simulink model "Tonneau"  (R2023b)
settings: Solver=VariableStepAuto  StartTime=0.0  StopTime=60  RelTol=1e-3
values from neighbouring files (symbols this model uses):
  p = @(t)  interp1(     [0, t_fin/30, t_fin/10, t_fin/5, 0.7*t_fin, 0.9*t_fin, t_fin],     [0, p_max/40, p_max*3/4,  p_max,     p_max,         0,     0],     t, 'pchip'  )    [ESERCIZIO_3_3.m]    (also in main.m = @(t)      interp1(          [0 t_fin/30 t_fin/10 t_fin/5 0.7; plotTrajectoryAndBody.m = patch('faces', F, 'vertices' ,Vb))
  PosE0 = [X0;Y0;Z0]    [ESERCIZIO_3_3.m]    (also in main.m = [0;0;0])
  Q0 = angle2quat(psi0, theta0, phi0)    [ESERCIZIO_3_3.m]    (also in main.m)
libraries: aerolibconvert2 x2, sharedtransform x2, SignalEditorBlockLib x2, aerolibutil x1
settings Model: Creator=Vincenzo  LastModifiedBy=agode
settings SolverCC: AlgebraicLoopSolver=TrustRegion
settings DebuggingCC: UnconnectedInputMsg=warning  UnconnectedOutputMsg=warning  UnconnectedLineMsg=warning  ArithmeticOperatorsInVariantConditions=warning
settings ModelReferenceCC: EnableRefExpFcnMdlSchedulingChecks=on
settings SFSimCC: SimUseLocalCustomCode=off  CustomCodeUndefinedFunction=UseInterfaceOnly
settings RTWCC: RTWUseLocalCustomCode=off

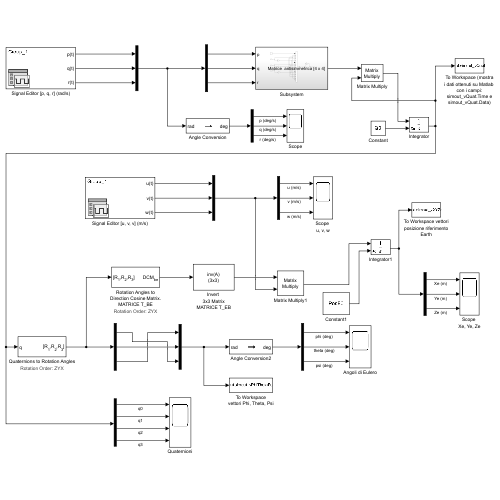
[thumbnail: Simulink's stored preview of the top-level diagram]
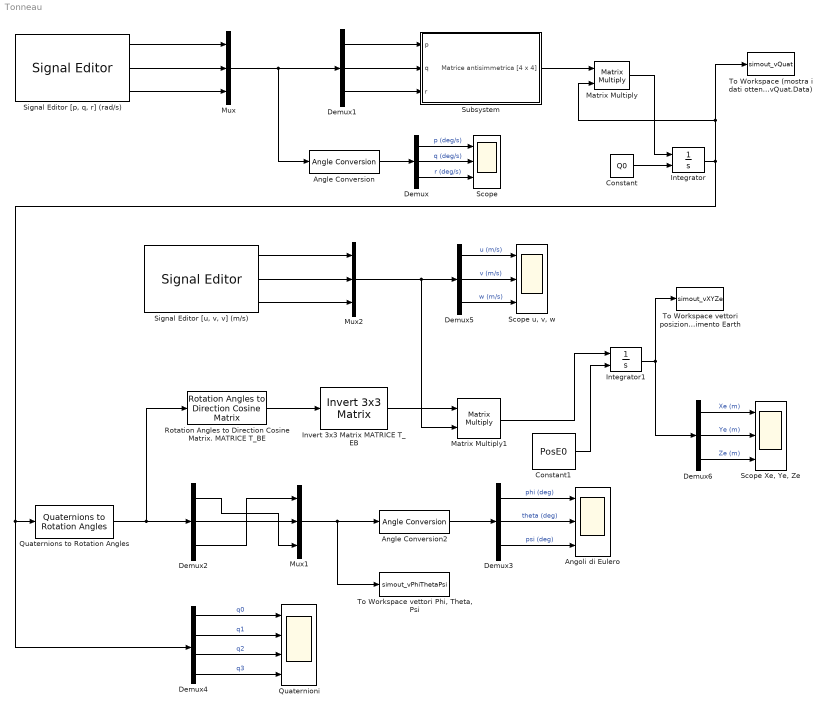
== system Tonneau ==
  Angle Conversion : aerolibconvert2/Angle Conversion  IU=rad  OU=deg
  Angle Conversion2 : aerolibconvert2/Angle Conversion  IU=rad  OU=deg
  Angoli di Eulero : Scope  NumInputPorts=3
  Constant : Constant  Value=Q0
  Constant1 : Constant  Value=PosE0
  Demux{,1..3,5..6} (6 alike) : Demux  Outputs=3
  Demux4 : Demux
  Integrator : Integrator  InitialConditionSource=external
  Integrator1 : Integrator  InitialConditionSource=external
  Invert 3x3 Matrix MATRICE T_EB : aerolibutil/Invert  3x3 Matrix
  Matrix Multiply : Product  Multiplication=Matrix(*)
  Matrix Multiply1 : Product  Multiplication=Matrix(*)
  Mux : Mux  Inputs=3
  Mux1 : Mux  Inputs=3
  Mux2 : Mux  Inputs=3
  Quaternioni : Scope  NumInputPorts=4
  Quaternions to Rotation Angles : sharedtransform/Quaternions to Rotation Angles  rotationOrder=ZYX  aMode=aMode
  Rotation Angles to Direction Cosine Matrix. MATRICE T_BE : sharedtransform/Rotation Angles to Direction Cosine Matrix  rotationOrder=ZYX  aMode=aMode
  Scope : Scope  NumInputPorts=3
  "Scope Xe, Ye, Ze" : Scope  NumInputPorts=3
  "Scope u, v, w" : Scope  NumInputPorts=3
  "Signal Editor [p, q, r] (rad/s)" : SignalEditorBlockLib/Signal Editor  FileName=signal_editor_pqr.mat  ActiveScenario=Dataset_pqr  ActiveSignal=p(t)  IsBus=off  OutputBusObjectStr=Bus: BusObject  SampleTime=0  ZeroCross=off  OutputAfterFinalValue=Setting to zero  Unit=inherit  PreserveSignalName=on  ApplySigPropsToAllScenarios=on  ApplySigPropsToAllSignals=on
  "Signal Editor [u, v, v] (m/s)" : SignalEditorBlockLib/Signal Editor  FileName=signal_editor_uvw.mat  ActiveScenario=Dataset_uvw  ActiveSignal=u(t)  IsBus=off  OutputBusObjectStr=Bus: BusObject  SampleTime=0  ZeroCross=off  OutputAfterFinalValue=Setting to zero  Unit=inherit  PreserveSignalName=on  ApplySigPropsToAllScenarios=on  ApplySigPropsToAllSignals=on
  Subsystem : Subsystem
  "To Workspace vettori Phi, Theta, Psi" : ToWorkspace  VariableName=simout_vPhiThetaPsi  SaveFormat=Timeseries  SampleTime=-1
  To Workspace (mostra i dati ottenuti su Matlab con i campi: simout_vQuat.Time e simout_vQuat.Data) : ToWorkspace  VariableName=simout_vQuat  SaveFormat=Timeseries  SampleTime=-1
  To Workspace vettori posizione riferimento Earth : ToWorkspace  VariableName=simout_vXYZe  SaveFormat=Timeseries  SampleTime=-1
  wires:
  Mux/1 -> Demux1/1, Angle Conversion/1
  Angle Conversion/1 -> Demux/1
  Demux/3 -> Scope/3  "r (deg/s)"
  Demux/2 -> Scope/2  "q (deg/s)"
  Demux/1 -> Scope/1  "p (deg/s)"
  "Signal Editor [p, q, r] (rad/s)"/1 -> Mux/1
  "Signal Editor [p, q, r] (rad/s)"/2 -> Mux/2
  "Signal Editor [p, q, r] (rad/s)"/3 -> Mux/3
  Demux1/2 -> Subsystem/2(q)
  Demux1/3 -> Subsystem/3(r)
  Demux1/1 -> Subsystem/1(p)
  Subsystem/1("Matrice antisimmetrica [4 x 4] ") -> Matrix Multiply/1
  Matrix Multiply/1 -> Integrator/1
  Constant/1 -> Integrator/2
  Integrator/1 -> Demux4/1, Quaternions to Rotation Angles/1, To Workspace (mostra i dati ottenuti su Matlab con i campi: simout_vQuat.Time e simout_vQuat.Data)/1, Matrix Multiply/2
  Quaternions to Rotation Angles/1 -> Rotation Angles to Direction Cosine Matrix. MATRICE T_BE/1, Demux2/1
  Demux2/3 -> Mux1/1
  Demux2/1 -> Mux1/3
  Demux2/2 -> Mux1/2
  Mux1/1 -> "To Workspace vettori Phi, Theta, Psi"/1, Angle Conversion2/1
  Angle Conversion2/1 -> Demux3/1
  Demux3/3 -> Angoli di Eulero/3  "psi (deg)"
  Demux3/2 -> Angoli di Eulero/2  "theta (deg)"
  Demux3/1 -> Angoli di Eulero/1  "phi (deg)"
  Demux4/1 -> Quaternioni/1  "q0"
  Demux4/2 -> Quaternioni/2  "q1"
  Demux4/3 -> Quaternioni/3  "q2"
  Demux4/4 -> Quaternioni/4  "q3"
  Rotation Angles to Direction Cosine Matrix. MATRICE T_BE/1 -> Invert 3x3 Matrix MATRICE T_EB/1
  "Signal Editor [u, v, v] (m/s)"/3 -> Mux2/3
  "Signal Editor [u, v, v] (m/s)"/1 -> Mux2/1
  "Signal Editor [u, v, v] (m/s)"/2 -> Mux2/2
  Demux5/1 -> "Scope u, v, w"/1  "u (m/s)"
  Demux5/2 -> "Scope u, v, w"/2  "v (m/s)"
  Demux5/3 -> "Scope u, v, w"/3  "w (m/s)"
  Mux2/1 -> Demux5/1, Matrix Multiply1/2
  Matrix Multiply1/1 -> Integrator1/1
  Constant1/1 -> Integrator1/2
  Demux6/2 -> "Scope Xe, Ye, Ze"/2  "Ye (m)"
  Integrator1/1 -> Demux6/1, To Workspace vettori posizione riferimento Earth/1
  Demux6/1 -> "Scope Xe, Ye, Ze"/1  "Xe (m)"
  Demux6/3 -> "Scope Xe, Ye, Ze"/3  "Ze (m)"
  Invert 3x3 Matrix MATRICE T_EB/1 -> Matrix Multiply1/1

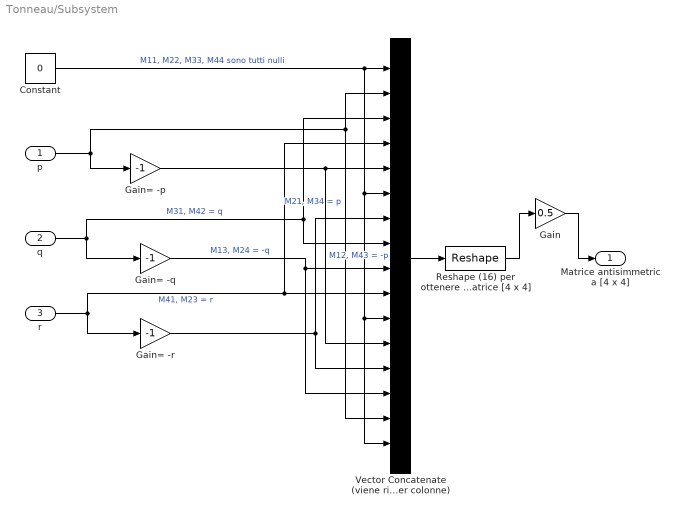
== system Tonneau/Subsystem ==
  p : Inport
  q : Inport  Port=2
  r : Inport  Port=3
  Constant : Constant  Value=0
  Gain : Gain  Gain=0.5
  Gain= -p : Gain  Gain=-1
  Gain= -q : Gain  Gain=-1
  Gain= -r : Gain  Gain=-1
  Reshape (16) per ottenere una matrice [4 x 4] : Reshape  OutputDimensionality=Customize  OutputDimensions=[4,4]
  Vector Concatenate (viene riempito per colonne) : Concatenate  NumInputs=16
  "Matrice antisimmetrica [4 x 4] " : Outport  VectorParamsAs1DForOutWhenUnconnected=off
  wires:
  Constant/1 -> Vector Concatenate (viene riempito per colonne)/16, Vector Concatenate (viene riempito per colonne)/11, Vector Concatenate (viene riempito per colonne)/6, Vector Concatenate (viene riempito per colonne)/1  "M11, M22, M33, M44 sono tutti nulli"
  p/1 -> Gain= -p/1, Vector Concatenate (viene riempito per colonne)/2, Vector Concatenate (viene riempito per colonne)/15  "M21, M34 = p"
  Gain= -p/1 -> Vector Concatenate (viene riempito per colonne)/12, Vector Concatenate (viene riempito per colonne)/5  "M12, M43 = -p"
  q/1 -> Gain= -q/1, Vector Concatenate (viene riempito per colonne)/8, Vector Concatenate (viene riempito per colonne)/3  "M31, M42 = q"
  Gain= -q/1 -> Vector Concatenate (viene riempito per colonne)/9, Vector Concatenate (viene riempito per colonne)/14  "M13, M24 = -q"
  r/1 -> Gain= -r/1, Vector Concatenate (viene riempito per colonne)/4, Vector Concatenate (viene riempito per colonne)/10  "M41, M23 = r"
  Gain= -r/1 -> Vector Concatenate (viene riempito per colonne)/13, Vector Concatenate (viene riempito per colonne)/7
  Vector Concatenate (viene riempito per colonne)/1 -> Reshape (16) per ottenere una matrice [4 x 4]/1
  Reshape (16) per ottenere una matrice [4 x 4]/1 -> Gain/1
  Gain/1 -> "Matrice antisimmetrica [4 x 4] "/1
